simulink model "Simulink_SS"  (R2020b)
settings: Solver=VariableStepAuto  StartTime=0.0  StopTime=3600  RelTol=1e-3
undefined symbols (not defined in the file): A, B, b, c, D, I, ic, N, P, sysSS, Ts
settings Model: Creator=jerem  LastModifiedBy=jerem

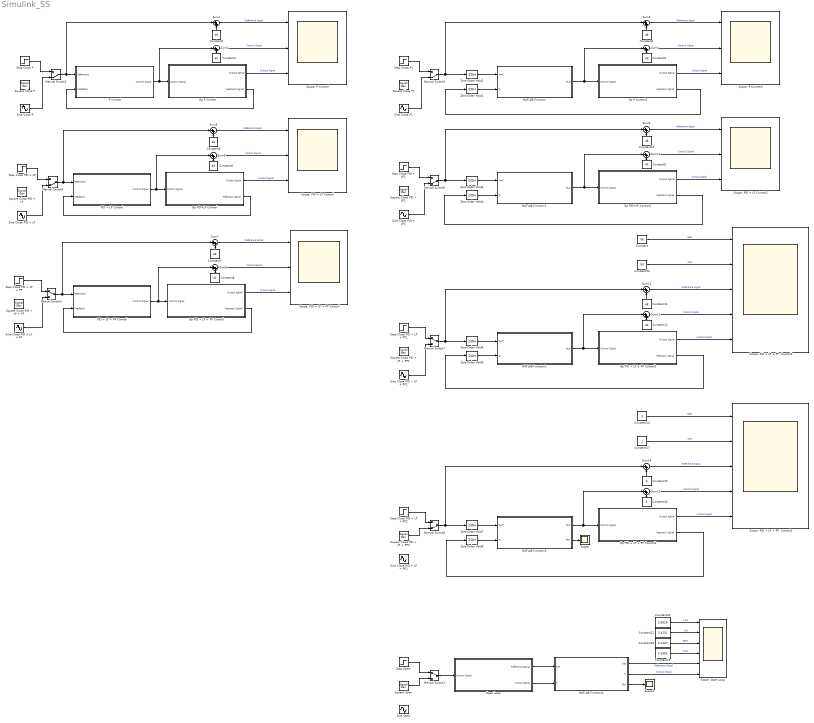
== system Simulink_SS ==
  Constant : Constant  Value=66
  Constant{1,3,5,8..9,12} (6 alike) : Constant  Value=40
  Constant{2,4,6..7,10..11} (6 alike) : Constant  Value=48
  Constant13 : Constant  Value=50
  Constant14 : Constant  Value=9
  Constant15 : Constant  Value=0
  Constant16 : Constant  Value=0
  Constant17 : Constant
  Constant18 : Constant  Value=3.1437
  Constant19 : Constant  Value=0.3493
  Constant20 : Constant  Value=3.5629
  Constant21 : Constant  Value=3.4231
  Gp P Control : Subsystem
  Gp P Control1 : Subsystem
  Gp PID + LP + PP Control : Subsystem
  Gp PID + LP + PP Control1 : Subsystem
  Gp PID + LP + PP Control2 : Subsystem
  Gp PID+LP Control : Subsystem
  Gp PID+LP Control1 : Subsystem
  MATLAB Function : MATLAB Function  TreatAsAtomicUnit=on
  MATLAB Function1 : MATLAB Function  TreatAsAtomicUnit=on
  MATLAB Function2 : MATLAB Function  TreatAsAtomicUnit=on
  MATLAB Function3 : MATLAB Function  TreatAsAtomicUnit=on
  MATLAB Function4 : MATLAB Function  TreatAsAtomicUnit=on
  Manual Switch1 : ManualSwitch
  Manual Switch{2..4,6,8} (5 alike) : ManualSwitch  CurrentSetting=0
  Manual Switch5 : ManualSwitch
  Manual Switch7 : ManualSwitch
  Open Loop : Subsystem
  P Control : Subsystem
  PID + LP + PP Control : Subsystem
  PID + LP Control : Subsystem
  Scope : Scope
  Scope1 : Scope
  Scope: Open Loop : Scope  NumInputPorts=6
  Scope: P Control : Scope  NumInputPorts=3
  Scope: P Control2 : Scope  NumInputPorts=3
  Scope: PID + LP + PP  Control1 : Scope  NumInputPorts=5
  Scope: PID + LP + PP  Control2 : Scope  NumInputPorts=5
  Scope: PID + LP + PP Control : Scope  NumInputPorts=3
  Scope: PID + LP Control : Scope  NumInputPorts=3
  Scope: PID + LP Control2 : Scope  NumInputPorts=3
  Sine Close P : Sin  Amplitude=20  Frequency=0.004  SampleTime=0
  Sine Close P1 : Sin  Amplitude=20  Frequency=0.004  SampleTime=0
  Sine Close PID + LP : Sin  Amplitude=20  Frequency=0.007  SampleTime=0
  Sine Close PID + LP + PP : Sin  Amplitude=10  Frequency=0.004  SampleTime=0
  Sine Close PID + LP + PP1 : Sin  Amplitude=10  Frequency=1/1800*6.28  SampleTime=0
  Sine Close PID + LP + PP2 : Sin  Amplitude=10  Frequency=1/1800*6.28  SampleTime=0
  Sine Close PID + LP1 : Sin  Amplitude=20  Frequency=0.007  SampleTime=0
  Sine Open : Sin  Amplitude=10  Frequency=1/1800*6.28  SampleTime=0
  Square Close P : SignalGenerator  WaveForm=square  Amplitude=20  Frequency=1/900
  Square Close P1 : SignalGenerator  WaveForm=square  Amplitude=20  Frequency=1/900
  Square Close PID + LP : SignalGenerator  WaveForm=square  Amplitude=20  Frequency=1/900
  Square Close PID + LP + PP : SignalGenerator  WaveForm=square  Amplitude=20  Frequency=1/900
  Square Close PID + LP + PP1 : SignalGenerator  WaveForm=square  Amplitude=20  Frequency=1/1800
  Square Close PID + LP + PP2 : SignalGenerator  WaveForm=square  Amplitude=10  Frequency=1/1800
  Square Close PID + LP1 : SignalGenerator  WaveForm=square  Amplitude=20  Frequency=1/900
  Square Open : SignalGenerator  WaveForm=square  Amplitude=10  Frequency=1/1800
  Step Close P : Step  After=20  SampleTime=Ts
  Step Close P1 : Step  After=20  SampleTime=Ts
  Step Close PID + LP : Step  After=20  SampleTime=Ts
  Step Close PID + LP + PP : Step  After=20  SampleTime=0.4
  Step Close PID + LP + PP1 : Step  After=10
  Step Close PID + LP + PP2 : Step  After=10
  Step Close PID + LP1 : Step  After=20  SampleTime=Ts
  Step Open : Step  After=10  SampleTime=1
  Sum{1..14} (14 alike) : Sum  Inputs=|++
  Zero-Order Hold{1..8} (8 alike) : ZeroOrderHold
  wires:
  Gp P Control/2(Feecback Sginal) -> P Control/2(Feedback)
  Constant1/1 -> Sum2/2
  Gp P Control/1(Output Sginal) -> Scope: P Control/3  "Output Signal"
  Constant2/1 -> Sum1/2
  Sum1/1 -> Scope: P Control/1  "Reference Signal"
  P Control/1(Control Signal) -> Sum2/1, Gp P Control/1(Control Signal)
  Manual Switch2/1 -> Sum1/1, P Control/1(Reference)
  Manual Switch1/1 -> Open Loop/1(Control Signal)
  Sum2/1 -> Scope: P Control/2  "Control Signal"
  Gp PID + LP + PP Control/2(Feecback Sginal) -> PID + LP + PP Control/2(Feedback)
  Sum8/1 -> Scope: PID + LP + PP Control/2  "Control Signal"
  Sum5/1 -> Scope: PID + LP Control/1  "Reference Signal"
  Sum7/1 -> Scope: PID + LP + PP Control/1  "Reference Signal"
  Sine Close PID + LP + PP/1 -> Manual Switch5/2
  Gp PID+LP Control/2(Feecback Sginal) -> PID + LP Control/2(Feedback)
  Constant7/1 -> Sum7/2
  Gp PID + LP + PP Control/1(Output Sginal) -> Scope: PID + LP + PP Control/3  "Output Signal"
  PID + LP + PP Control/1(Control Signal) -> Sum8/1, Gp PID + LP + PP Control/1(Control Signal)
  Gp PID+LP Control/1(Output Sginal) -> Scope: PID + LP Control/3  "Output Signal"
  Manual Switch5/1 -> PID + LP + PP Control/1(Reference), Sum7/1
  Step Close PID + LP + PP/1 -> Manual Switch5/1
  Constant6/1 -> Sum5/2
  Manual Switch4/1 -> Sum5/1, PID + LP Control/1(Reference)
  Constant8/1 -> Sum8/2
  PID + LP Control/1(Control Signal) -> Sum6/1, Gp PID+LP Control/1(Control Signal)
  Sum6/1 -> Scope: PID + LP Control/2  "Control Signal"
  Constant5/1 -> Sum6/2
  Sum11/1 -> Scope: PID + LP + PP  Control2/4  "Control Signal"
  Constant3/1 -> Sum4/2
  Constant10/1 -> Sum9/2
  Constant9/1 -> Sum10/2
  Sum9/1 -> Scope: PID + LP Control2/1  "Reference Signal"
  Sum10/1 -> Scope: PID + LP Control2/2  "Control Signal"
  Gp PID+LP Control1/1(Output Sginal) -> Scope: PID + LP Control2/3  "Output Signal"
  Gp PID+LP Control1/2(Feecback Sginal) -> Zero-Order Hold4/1
  Gp P Control1/1(Output Sginal) -> Scope: P Control2/3  "Output Signal"
  Sum3/1 -> Scope: P Control2/1  "Reference Signal"
  Gp P Control1/2(Feecback Sginal) -> Zero-Order Hold1/1
  Manual Switch6/1 -> Sum9/1, Zero-Order Hold3/1
  Constant4/1 -> Sum3/2
  Manual Switch7/1 -> Sum12/1, Zero-Order Hold5/1
  Gp PID + LP + PP Control1/2(Feecback Sginal) -> Zero-Order Hold6/1
  Manual Switch3/1 -> Sum3/1, Zero-Order Hold2/1
  MATLAB Function1/1(fout) -> Sum10/1, Gp PID+LP Control1/1(Control Signal)
  Gp PID + LP + PP Control1/1(Output Sginal) -> Scope: PID + LP + PP  Control2/5  "Output Signal"
  Sum12/1 -> Scope: PID + LP + PP  Control2/3  "Reference Signal"
  MATLAB Function2/1(fout) -> Gp PID + LP + PP Control1/1(Control Signal), Sum11/1
  Sum4/1 -> Scope: P Control2/2  "Control Signal"
  MATLAB Function/1(fout) -> Gp P Control1/1(Control Signal), Sum4/1
  Constant12/1 -> Sum11/2
  Constant11/1 -> Sum12/2
  Step Close PID + LP + PP1/1 -> Manual Switch7/1
  Step Close PID + LP/1 -> Manual Switch4/1
  Sine Close PID + LP/1 -> Manual Switch4/2
  Step Close PID + LP1/1 -> Manual Switch6/1
  Sine Close PID + LP1/1 -> Manual Switch6/2
  Step Close P1/1 -> Manual Switch3/1
  Sine Close P1/1 -> Manual Switch3/2
  Step Close P/1 -> Manual Switch2/1
  Sine Close P/1 -> Manual Switch2/2
  Step Open/1 -> Manual Switch1/1
  Zero-Order Hold1/1 -> MATLAB Function/2(fy)
  Zero-Order Hold2/1 -> MATLAB Function/1(fref)
  Zero-Order Hold3/1 -> MATLAB Function1/1(fref)
  Zero-Order Hold4/1 -> MATLAB Function1/2(fy)
  Zero-Order Hold5/1 -> MATLAB Function2/1(fref)
  Zero-Order Hold6/1 -> MATLAB Function2/2(fy)
  Sine Close PID + LP + PP1/1 -> Manual Switch7/2
  Constant/1 -> Scope: PID + LP + PP  Control2/1  "90%"
  Constant13/1 -> Scope: PID + LP + PP  Control2/2  "10%"
  Step Close PID + LP + PP2/1 -> Manual Switch8/1
  Constant16/1 -> Sum13/2
  Sum14/1 -> Scope: PID + LP + PP  Control1/3  "Reference Signal"
  Gp PID + LP + PP Control2/1(Output Sginal) -> Scope: PID + LP + PP  Control1/5  "Output Signal"
  Constant14/1 -> Scope: PID + LP + PP  Control1/1  "90%"
  MATLAB Function3/1(fout) -> Sum13/1, Gp PID + LP + PP Control2/1(Control Signal)
  Constant15/1 -> Sum14/2
  Constant17/1 -> Scope: PID + LP + PP  Control1/2  "10%"
  Sum13/1 -> Scope: PID + LP + PP  Control1/4  "Control Signal"
  Zero-Order Hold7/1 -> MATLAB Function3/1(fref)
  Manual Switch8/1 -> Sum14/1, Zero-Order Hold7/1
  Zero-Order Hold8/1 -> MATLAB Function3/2(fy)
  Gp PID + LP + PP Control2/2(Feecback Sginal) -> Zero-Order Hold8/1
  MATLAB Function3/2(fErr) -> Scope/1
  Square Close PID + LP + PP2/1 -> Manual Switch8/2
  Open Loop/2(Output Sginal) -> MATLAB Function4/2("fy ")
  Open Loop/1(Reference Sginal) -> MATLAB Function4/1("fref ")
  MATLAB Function4/3(fErr) -> Scope1/1
  Constant19/1 -> Scope: Open Loop/4  "10%"
  MATLAB Function4/1(fref) -> Scope: Open Loop/5  "Reference Signal"
  Constant18/1 -> Scope: Open Loop/3  "90%"
  MATLAB Function4/2(fy) -> Scope: Open Loop/6  "Output Signal"
  Square Open/1 -> Manual Switch1/2
  Constant21/1 -> Scope: Open Loop/2  "-2%"
  Constant20/1 -> Scope: Open Loop/1  "+2%"

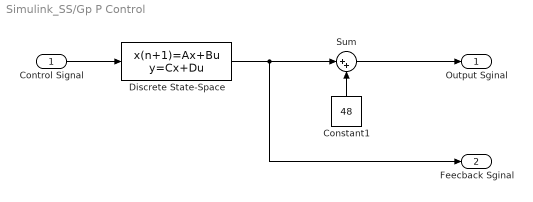
== system Simulink_SS/Gp P Control ==
  Control Signal : Inport
  Constant1 : Constant  Value=48
  Discrete State-Space : DiscreteStateSpace  A=sysSS.A  B=sysSS.B  C=sysSS.C  D=sysSS.D  InitialCondition=ic  SampleTime=Ts
  Sum : Sum  Inputs=|++
  Output Sginal : Outport
  Feecback Sginal : Outport  Port=2
  wires:
  Discrete State-Space/1 -> Feecback Sginal/1, Sum/1
  Sum/1 -> Output Sginal/1
  Constant1/1 -> Sum/2
  Control Signal/1 -> Discrete State-Space/1

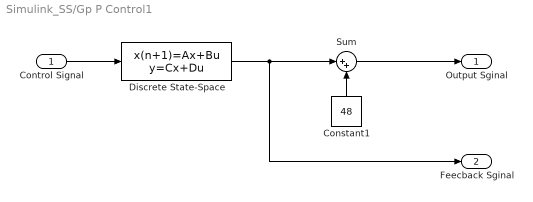
== system Simulink_SS/Gp P Control1 ==
  Control Signal : Inport
  Constant1 : Constant  Value=48
  Discrete State-Space : DiscreteStateSpace  A=sysSS.A  B=sysSS.B  C=sysSS.C  D=sysSS.D  InitialCondition=ic  SampleTime=Ts
  Sum : Sum  Inputs=|++
  Output Sginal : Outport
  Feecback Sginal : Outport  Port=2
  wires:
  Discrete State-Space/1 -> Feecback Sginal/1, Sum/1
  Sum/1 -> Output Sginal/1
  Constant1/1 -> Sum/2
  Control Signal/1 -> Discrete State-Space/1

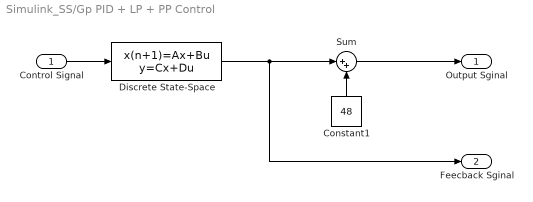
== system Simulink_SS/Gp PID + LP + PP Control ==
  Control Signal : Inport
  Constant1 : Constant  Value=48
  Discrete State-Space : DiscreteStateSpace  A=sysSS.A  B=sysSS.B  C=sysSS.C  D=sysSS.D  InitialCondition=ic  SampleTime=Ts
  Sum : Sum  Inputs=|++
  Output Sginal : Outport
  Feecback Sginal : Outport  Port=2
  wires:
  Discrete State-Space/1 -> Feecback Sginal/1, Sum/1
  Sum/1 -> Output Sginal/1
  Constant1/1 -> Sum/2
  Control Signal/1 -> Discrete State-Space/1

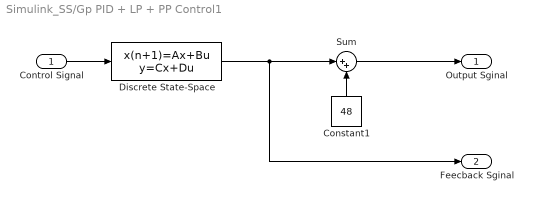
== system Simulink_SS/Gp PID + LP + PP Control1 ==
  Control Signal : Inport
  Constant1 : Constant  Value=48
  Discrete State-Space : DiscreteStateSpace  A=sysSS.A  B=sysSS.B  C=sysSS.C  D=sysSS.D  InitialCondition=ic  SampleTime=Ts
  Sum : Sum  Inputs=|++
  Output Sginal : Outport
  Feecback Sginal : Outport  Port=2
  wires:
  Discrete State-Space/1 -> Feecback Sginal/1, Sum/1
  Sum/1 -> Output Sginal/1
  Constant1/1 -> Sum/2
  Control Signal/1 -> Discrete State-Space/1

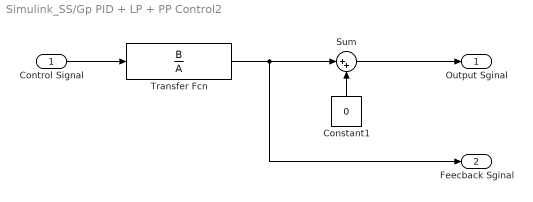
== system Simulink_SS/Gp PID + LP + PP Control2 ==
  Control Signal : Inport
  Constant1 : Constant  Value=0
  Sum : Sum  Inputs=|++
  Transfer Fcn : TransferFcn  Numerator=B  Denominator=A
  Output Sginal : Outport
  Feecback Sginal : Outport  Port=2
  wires:
  Transfer Fcn/1 -> Feecback Sginal/1, Sum/1
  Sum/1 -> Output Sginal/1
  Constant1/1 -> Sum/2
  Control Signal/1 -> Transfer Fcn/1

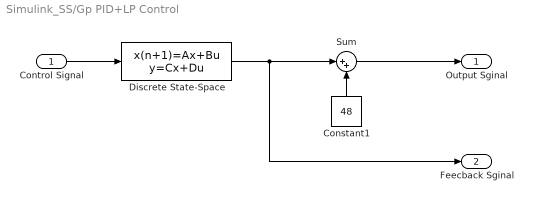
== system Simulink_SS/Gp PID+LP Control ==
  Control Signal : Inport
  Constant1 : Constant  Value=48
  Discrete State-Space : DiscreteStateSpace  A=sysSS.A  B=sysSS.B  C=sysSS.C  D=sysSS.D  InitialCondition=ic  SampleTime=Ts
  Sum : Sum  Inputs=|++
  Output Sginal : Outport
  Feecback Sginal : Outport  Port=2
  wires:
  Discrete State-Space/1 -> Feecback Sginal/1, Sum/1
  Sum/1 -> Output Sginal/1
  Constant1/1 -> Sum/2
  Control Signal/1 -> Discrete State-Space/1

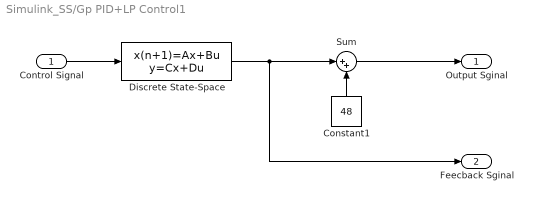
== system Simulink_SS/Gp PID+LP Control1 ==
  Control Signal : Inport
  Constant1 : Constant  Value=48
  Discrete State-Space : DiscreteStateSpace  A=sysSS.A  B=sysSS.B  C=sysSS.C  D=sysSS.D  InitialCondition=ic  SampleTime=Ts
  Sum : Sum  Inputs=|++
  Output Sginal : Outport
  Feecback Sginal : Outport  Port=2
  wires:
  Discrete State-Space/1 -> Feecback Sginal/1, Sum/1
  Sum/1 -> Output Sginal/1
  Constant1/1 -> Sum/2
  Control Signal/1 -> Discrete State-Space/1

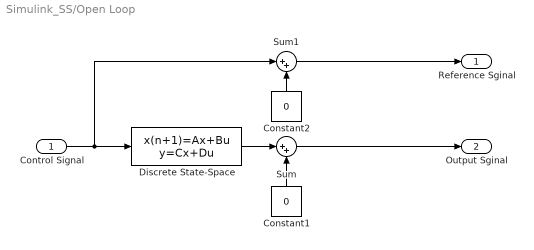
== system Simulink_SS/Open Loop ==
  Control Signal : Inport
  Constant1 : Constant  Value=0
  Constant2 : Constant  Value=0
  Discrete State-Space : DiscreteStateSpace  A=sysSS.A  B=sysSS.B  C=sysSS.C  D=sysSS.D  InitialCondition=ic  SampleTime=Ts
  Sum : Sum  Inputs=|++
  Sum1 : Sum  Inputs=|++
  Reference Sginal : Outport
  Output Sginal : Outport  Port=2
  wires:
  Discrete State-Space/1 -> Sum/1
  Sum/1 -> Output Sginal/1
  Constant2/1 -> Sum1/2
  Constant1/1 -> Sum/2
  Control Signal/1 -> Sum1/1, Discrete State-Space/1
  Sum1/1 -> Reference Sginal/1

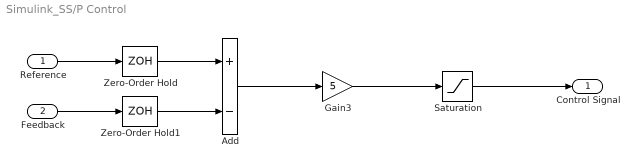
== system Simulink_SS/P Control ==
  Reference : Inport
  Feedback : Inport  Port=2
  Add : Sum  Inputs=+-
  Gain3 : Gain  Gain=5
  Saturation : Saturate  UpperLimit=60  LowerLimit=-40
  Zero-Order Hold : ZeroOrderHold
  Zero-Order Hold1 : ZeroOrderHold
  Control Signal : Outport
  wires:
  Reference/1 -> Zero-Order Hold/1
  Feedback/1 -> Zero-Order Hold1/1
  Saturation/1 -> Control Signal/1
  Zero-Order Hold/1 -> Add/1
  Add/1 -> Gain3/1
  Gain3/1 -> Saturation/1
  Zero-Order Hold1/1 -> Add/2

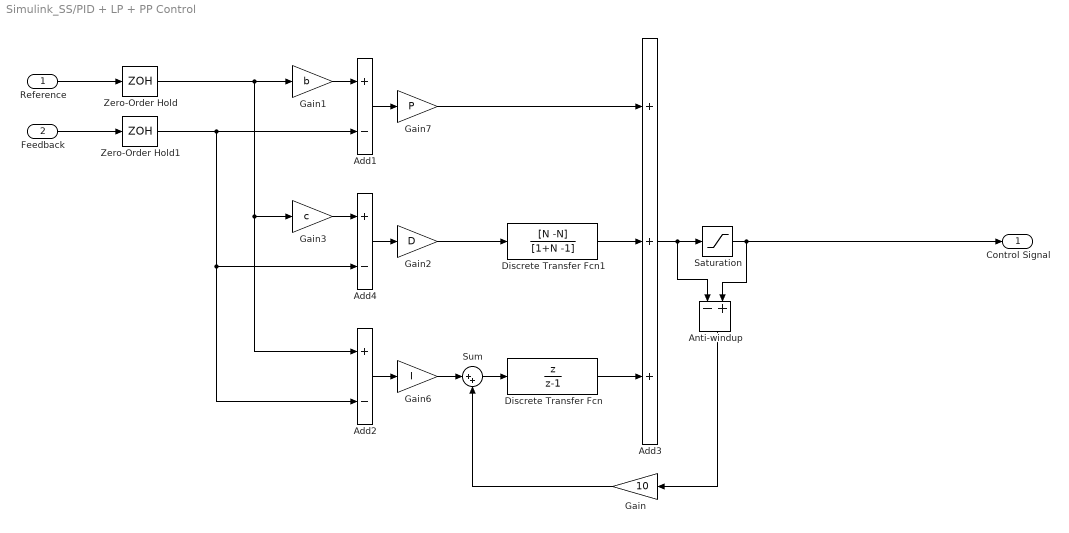
== system Simulink_SS/PID + LP + PP Control ==
  Reference : Inport
  Feedback : Inport  Port=2
  Add1 : Sum  Inputs=+-
  Add2 : Sum  Inputs=+-
  Add3 : Sum  Inputs=+++
  Add4 : Sum  Inputs=+-
  Anti-windup : Sum  Inputs=-+
  Discrete Transfer Fcn : DiscreteTransferFcn  Numerator=[1 0]  Denominator=[1 -1]  SampleTime=Ts
  Discrete Transfer Fcn1 : DiscreteTransferFcn  Numerator=[N -N]  Denominator=[1+N -1]  SampleTime=Ts
  Gain : Gain  Gain=10
  Gain1 : Gain  Gain=b
  Gain2 : Gain  Gain=D
  Gain3 : Gain  Gain=c
  Gain6 : Gain  Gain=I
  Gain7 : Gain  Gain=P
  Saturation : Saturate  UpperLimit=60  LowerLimit=-40
  Sum : Sum  Inputs=|++
  Zero-Order Hold : ZeroOrderHold
  Zero-Order Hold1 : ZeroOrderHold
  Control Signal : Outport
  wires:
  Gain1/1 -> Add1/1
  Zero-Order Hold/1 -> Gain1/1, Gain3/1, Add2/1
  Feedback/1 -> Zero-Order Hold1/1
  Reference/1 -> Zero-Order Hold/1
  Anti-windup/1 -> Gain/1
  Saturation/1 -> Anti-windup/2, Control Signal/1
  Gain/1 -> Sum/2
  Add3/1 -> Saturation/1, Anti-windup/1
  Gain3/1 -> Add4/1
  Discrete Transfer Fcn1/1 -> Add3/2
  Add1/1 -> Gain7/1
  Gain7/1 -> Add3/1
  Add4/1 -> Gain2/1
  Gain2/1 -> Discrete Transfer Fcn1/1
  Add2/1 -> Gain6/1
  Discrete Transfer Fcn/1 -> Add3/3
  Sum/1 -> Discrete Transfer Fcn/1
  Gain6/1 -> Sum/1
  Zero-Order Hold1/1 -> Add1/2, Add4/2, Add2/2

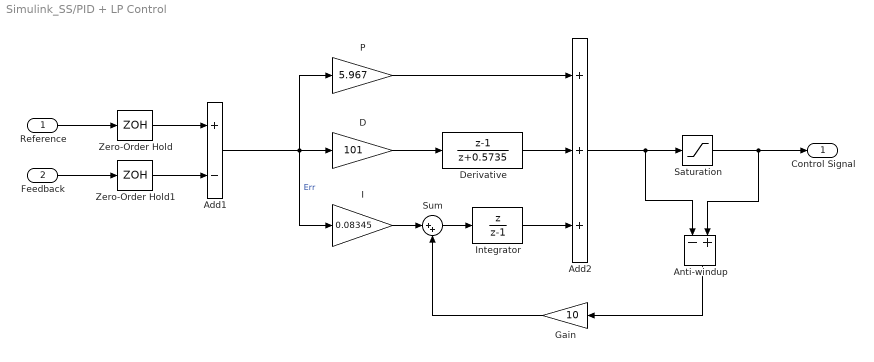
== system Simulink_SS/PID + LP Control ==
  Reference : Inport
  Feedback : Inport  Port=2
  Add1 : Sum  Inputs=+-
  Add2 : Sum  Inputs=+++
  Anti-windup : Sum  Inputs=-+
  D : Gain  Gain=101
  Derivative : DiscreteTransferFcn  Numerator=[1 -1]  Denominator=[1 0.5735]  SampleTime=Ts
  Gain : Gain  Gain=10
  I : Gain  Gain=0.08345
  Integrator : DiscreteTransferFcn  Numerator=[1 0]  Denominator=[1 -1]  SampleTime=Ts
  P : Gain  Gain=5.967
  Saturation : Saturate  UpperLimit=60  LowerLimit=-40
  Sum : Sum  Inputs=|++
  Zero-Order Hold : ZeroOrderHold
  Zero-Order Hold1 : ZeroOrderHold
  Control Signal : Outport
  wires:
  Add2/1 -> Anti-windup/1, Saturation/1
  Saturation/1 -> Anti-windup/2, Control Signal/1
  Zero-Order Hold/1 -> Add1/1
  Add1/1 -> I/1, D/1, P/1  "Err"
  Integrator/1 -> Add2/3
  P/1 -> Add2/1
  Anti-windup/1 -> Gain/1
  I/1 -> Sum/1
  Gain/1 -> Sum/2
  Sum/1 -> Integrator/1
  Reference/1 -> Zero-Order Hold/1
  Feedback/1 -> Zero-Order Hold1/1
  D/1 -> Derivative/1
  Derivative/1 -> Add2/2
  Zero-Order Hold1/1 -> Add1/2

== matlab function Simulink_SS/MATLAB Function1 ==
  data: fref input; fout output; fy input
function fout = fcn(fref, fy)
%%%%%%%%%%%%%%%%%%%%%%%%%%%%%%%%%%%%%%%%%%%%%%%%%%%%%%%
% PID + LP for SS
% Input : fref - reference signal
%         fy   - feedback signal
% Output: fout - control signal
%%%%%%%%%%%%%%%%%%%%%%%%%%%%%%%%%%%%%%%%%%%%%%%%%%%%%%%
% Variable Initialisation
persistent fD_prev fI_prev fIA_prev fErr_prev fant;
N = 0.5735; % Low pass filter value
Ts = 1;    % Sampling time
P = 6;
D = 101;
I = 0.083;
Kant = 1;

if isempty(fD_prev)
    fD_prev = 0;
    fI_prev = 0;
    fIA_prev = 0;
    fErr_prev = 0;
    fant = 0;
end

fErr = fref - fy;

% P
fP = P*(fref - fy);
% D
fD = (D/Ts)*(fErr - fErr_prev) - (N*fD_prev);
% I
fI = fI_prev + fErr*I*Ts;
% Kant = 10
fIA = fIA_prev + Kant*fant;

fsum = fP + fD + fI + fIA;

if fsum > 60
    fout = 60;
elseif fsum < (-40)
    fout = -40;
else
    fout = fsum;
end

% Update values
fErr_prev = fErr;
fD_prev = fD;
fI_prev = fI;
fIA_prev = fIA;
fant = fout - fsum;
end

== matlab function Simulink_SS/MATLAB Function ==
  data: fref input; fout output; fy input
function fout = fcn(fref, fy)
%%%%%%%%%%%%%%%%%%%%%%%%%%%%%%%%%%%%%%%%%%%%%%%%%%%%%%%
% P for SS
% Input : fref - reference signal
%         fy   - feedback signal
% Output: fout - control signal
%%%%%%%%%%%%%%%%%%%%%%%%%%%%%%%%%%%%%%%%%%%%%%%%%%%%%%%
P = 5;
fp = P*(fref - fy);

if fp > 60
    fout = 60;
elseif fp < (-40)
    fout = -40;
else
    fout = fp;
end
end

== matlab function Simulink_SS/MATLAB Function2 ==
  data: fref input; fout output; fy input
function fout = fcn(fref, fy)
%%%%%%%%%%%%%%%%%%%%%%%%%%%%%%%%%%%%%%%%%%%%%%%%%%%%%%%
% PID + LP + PP for SS
% Input : fref - reference signal
%         fy   - feedback signal
% Output: fout - control signal
%%%%%%%%%%%%%%%%%%%%%%%%%%%%%%%%%%%%%%%%%%%%%%%%%%%%%%%
% Variable Initialisation
persistent fD_prev fI_prev fIA_prev fDErr_prev fant;
Ts = 1;    % Sampling time
% P = 6.071;
% I = 0.07238;
% D = 122.1;
% N = 0.5735;
% b = 1;
% c = 1;

% P = 7.185;
% I = 0.1006;
% D = 126.3;
% N = 0.5253;
% b = 0.04062;
% c = 0.0007977;

P = 2.347;
I = 0.02086;
D = 2.894;
N = 0.9731;
b = 1;
c = 1;
Kant = 0.01;

if isempty(fD_prev)
    fD_prev = 0;
    fI_prev = 0;
    fIA_prev = 0;
    fDErr_prev = 0;
    fant = 0;
    
end

fErr = fref - fy;
fDErr = fref*c - fy;

% P
fP = P*(b*fref - fy);
% D
fD = D*N*(fDErr - fDErr_prev) + fD_prev/(1+N*Ts);
% I
fI = fI_prev + fErr*I*Ts;
% Kant = 10
fIA = fIA_prev + Kant*fant;

fsum = fP + fD + fI + fIA;

if fsum > 60
    fout = 60;
elseif fsum < (-40)
    fout = -40;
else
    fout = fsum;
end

% Update values
fDErr_prev = fDErr;
fD_prev = fD;
fI_prev = fI;
fIA_prev = fIA;
fant = fout - fsum;
end

== matlab function Simulink_SS/MATLAB Function3 ==
  data: fref input; fout output; fy input; fErr output
function [fout, fErr] = fcn(fref, fy)
%%%%%%%%%%%%%%%%%%%%%%%%%%%%%%%%%%%%%%%%%%%%%%%%%%%%%%%
% PID + LP + PP for SS
% Input : fref - reference signal
%         fy   - feedback signal
% Output: fout - control signal
%%%%%%%%%%%%%%%%%%%%%%%%%%%%%%%%%%%%%%%%%%%%%%%%%%%%%%%
% Variable Initialisation
persistent fD_prev fI_prev fIA_prev fDErr_prev fant;
Ts = 1;    % Sampling time

% ---- Rise Time 120 sec
% P = 5.656;
% I = 0.07951;
% D = 6.479;
% N = 0.5348;
% b = 0.017;
% c = 3.441e-05;

% Blane Rise Time 119.6 sec
P = 3.4044;
I = 0.0438;
D = 55.0446;
N = 0.0652;
b = 0.9023;
c = 0.5979;

Kant = 0.06;

if isempty(fD_prev)
    fD_prev = 0;
    fI_prev = 0;
    fIA_prev = 0;
    fDErr_prev = 0;
    fant = 0;
    
end

fErr = fref - fy;
fDErr = fref*c - fy;

% P
fP = P*(b*fref - fy);
% D
fD = (D*N*(fDErr - fDErr_prev) + fD_prev)/(1+N*Ts);
% I
fI = fI_prev + fErr*I*Ts;
% Kant = 10
fIA = fIA_prev + Kant*fant;

fsum = fP + fD + fI + fIA;

if fsum > 60
    fout = 60;
elseif fsum < (-40)
    fout = -40;
else
    fout = fsum;
end

% Update values
fDErr_prev = fDErr;
fD_prev = fD;
fI_prev = fI;
fIA_prev = fIA;
fant = fout - fsum;
end

== matlab function Simulink_SS/MATLAB Function4 ==
  data: fref input; fref output; fy output; fy input; fErr output
function [fref, fy, fErr] = fcn(fref, fy)
fErr = fref - fy;
end
